simulink model "ALU"  (R2022a)
settings: Solver=VariableStepAuto  StartTime=0.0  StopTime=10.0  RelTol=1e-3
settings Model: Creator=cuomo  LastModifiedBy=cuomo

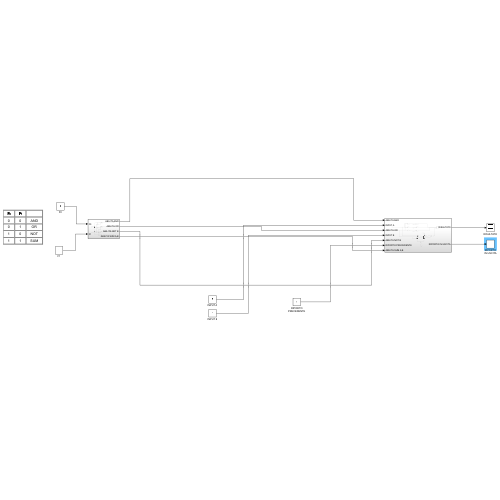
[thumbnail: Simulink's stored preview of the top-level diagram]
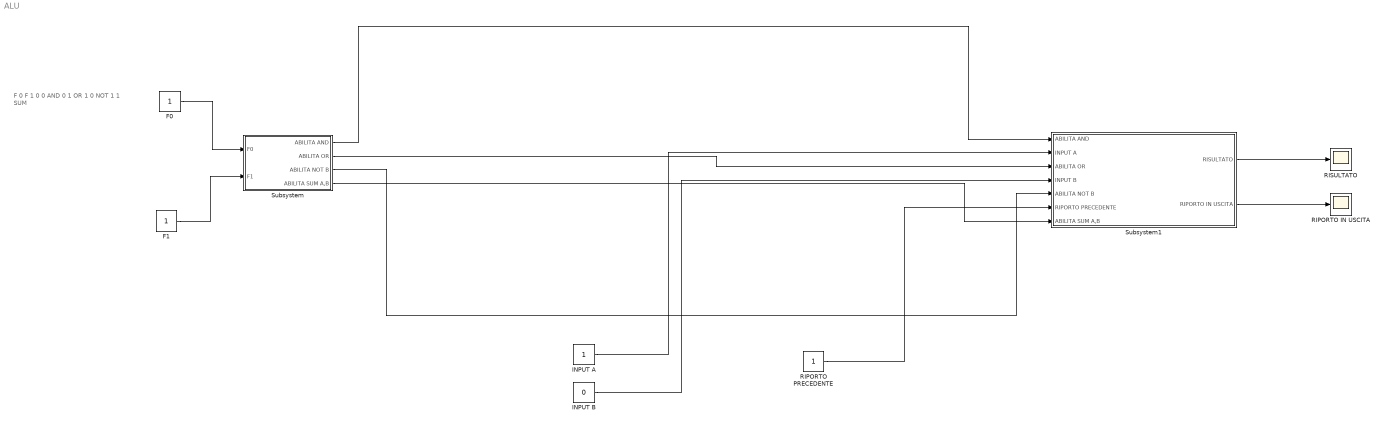
== system ALU ==
  note: F 0
      | F 1
      |
      | 0
      | 0
      | AND
      |
      | 0
      | 1
      | OR
      |
      | 1
      | 0
      | NOT
      |
      | 1
      | 1
      | SUM
  F0 : Constant
  F1 : Constant
  INPUT A : Constant
  INPUT B : Constant  Value=0
  RIPORTO IN USCITA : Scope
  RIPORTO PRECEDENTE : Constant
  RISULTATO : Scope
  Subsystem : Subsystem
  Subsystem1 : Subsystem
  wires:
  F1/1 -> Subsystem/2(F1)
  Subsystem/3(ABILITA NOT B) -> Subsystem1/5(ABILITA NOT B)
  Subsystem/4(ABILITA SUM A,B) -> Subsystem1/7(ABILITA SUM A,B)
  Subsystem/2(ABILITA OR) -> Subsystem1/3(ABILITA OR)
  RIPORTO PRECEDENTE/1 -> Subsystem1/6(RIPORTO PRECEDENTE)
  Subsystem/1(ABILITA AND) -> Subsystem1/1(ABILITA AND)
  INPUT A/1 -> Subsystem1/2(INPUT A)
  Subsystem1/1(RISULTATO) -> RISULTATO/1
  INPUT B/1 -> Subsystem1/4(INPUT B)
  Subsystem1/2(RIPORTO IN USCITA) -> RIPORTO IN USCITA/1
  F0/1 -> Subsystem/1(F0)

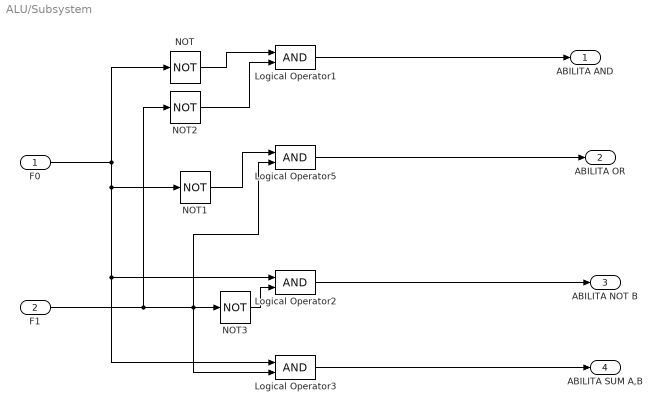
== system ALU/Subsystem ==
  F0 : Inport
  F1 : Inport  Port=2
  Logical Operator{1..3,5} (4 alike) : Logic  IconShape=distinctive  AllPortsSameDT=off  OutDataTypeStr=boolean
  NOT{,1..3} (4 alike) : Logic  Operator=NOT  IconShape=distinctive  AllPortsSameDT=off  OutDataTypeStr=boolean
  ABILITA AND : Outport
  ABILITA OR : Outport  Port=2
  ABILITA NOT B : Outport  Port=3
  ABILITA SUM A,B : Outport  Port=4
  wires:
  NOT2/1 -> Logical Operator1/2
  F0/1 -> Logical Operator3/1, Logical Operator2/1, NOT1/1, NOT/1
  F1/1 -> NOT2/1, Logical Operator3/2, Logical Operator5/2, NOT3/1
  Logical Operator5/1 -> ABILITA OR/1
  Logical Operator2/1 -> ABILITA NOT B/1
  NOT3/1 -> Logical Operator2/2
  Logical Operator3/1 -> ABILITA SUM A,B/1
  NOT1/1 -> Logical Operator5/1
  Logical Operator1/1 -> ABILITA AND/1
  NOT/1 -> Logical Operator1/1

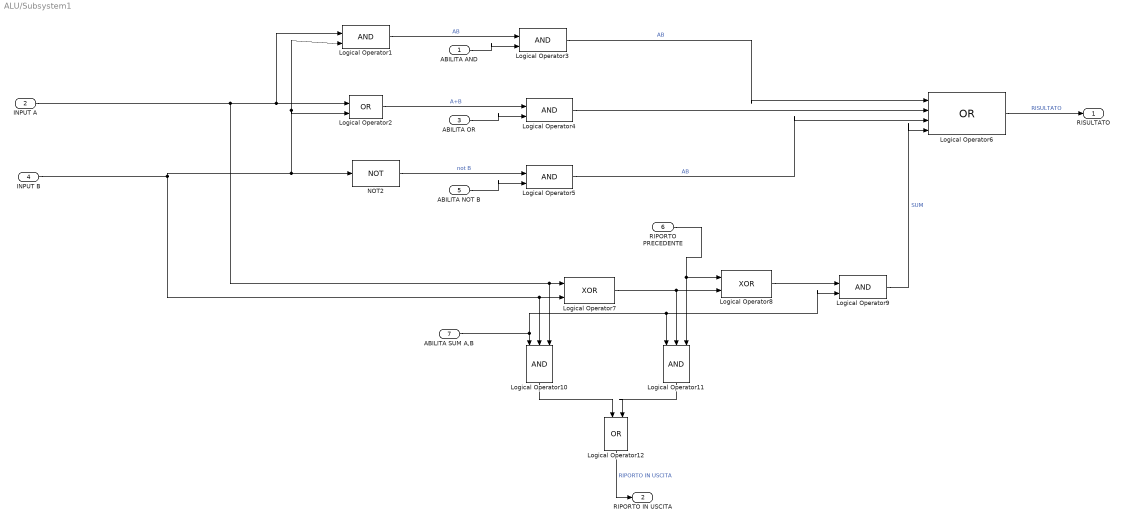
== system ALU/Subsystem1 ==
  ABILITA AND : Inport
  INPUT A : Inport  Port=2
  ABILITA OR : Inport  Port=3
  INPUT B : Inport  Port=4
  ABILITA NOT B : Inport  Port=5
  RIPORTO PRECEDENTE : Inport  Port=6
  ABILITA SUM A,B : Inport  Port=7
  Logical Operator{1,3..5,9} (5 alike) : Logic  IconShape=distinctive  AllPortsSameDT=off  OutDataTypeStr=boolean
  Logical Operator10 : Logic  Inputs=3  IconShape=distinctive  AllPortsSameDT=off  OutDataTypeStr=boolean
  Logical Operator11 : Logic  Inputs=3  IconShape=distinctive  AllPortsSameDT=off  OutDataTypeStr=boolean
  Logical Operator12 : Logic  Operator=OR  IconShape=distinctive  AllPortsSameDT=off  OutDataTypeStr=boolean
  Logical Operator2 : Logic  Operator=OR  IconShape=distinctive  AllPortsSameDT=off  OutDataTypeStr=boolean
  Logical Operator6 : Logic  Operator=OR  Inputs=4  IconShape=distinctive  AllPortsSameDT=off  OutDataTypeStr=boolean
  Logical Operator7 : Logic  Operator=XOR  IconShape=distinctive  AllPortsSameDT=off  OutDataTypeStr=boolean
  Logical Operator8 : Logic  Operator=XOR  IconShape=distinctive  AllPortsSameDT=off  OutDataTypeStr=boolean
  NOT2 : Logic  Operator=NOT  IconShape=distinctive  AllPortsSameDT=off  OutDataTypeStr=boolean
  RISULTATO : Outport
  RIPORTO IN USCITA : Outport  Port=2
  wires:
  ABILITA AND/1 -> Logical Operator3/2
  Logical Operator7/1 -> Logical Operator11/2, Logical Operator8/2
  RIPORTO PRECEDENTE/1 -> Logical Operator8/1, Logical Operator11/3
  Logical Operator12/1 -> RIPORTO IN USCITA/1  "RIPORTO IN USCITA"
  NOT2/1 -> Logical Operator5/1  "not B"
  Logical Operator3/1 -> Logical Operator6/1  "AB"
  Logical Operator5/1 -> Logical Operator6/3  "AB"
  INPUT A/1 -> Logical Operator1/1, Logical Operator2/1, Logical Operator10/3, Logical Operator7/1
  INPUT B/1 -> Logical Operator1/2, Logical Operator2/2, NOT2/1, Logical Operator10/2, Logical Operator7/2
  Logical Operator2/1 -> Logical Operator4/1  "A+B"
  ABILITA SUM A,B/1 -> Logical Operator11/1, Logical Operator9/2, Logical Operator10/1
  Logical Operator9/1 -> Logical Operator6/4  "SUM"
  ABILITA NOT B/1 -> Logical Operator5/2
  Logical Operator11/1 -> Logical Operator12/2
  Logical Operator10/1 -> Logical Operator12/1
  ABILITA OR/1 -> Logical Operator4/2
  Logical Operator8/1 -> Logical Operator9/1
  Logical Operator6/1 -> RISULTATO/1  "RISULTATO"
  Logical Operator1/1 -> Logical Operator3/1  "AB"
  Logical Operator4/1 -> Logical Operator6/2
